simulink model "Joystick"  (R2018a)
settings: Solver=FixedStepDiscrete  StartTime=0.0  StopTime=inf  RelTol=1e-3  EnableMultiTasking=on
libraries: simulink x5, CustomLibrary x5
settings Model: SimulationMode=external  ExtModeTrigDuration=2  Creator=jonathancoulter  LastModifiedBy=jonathancoulter
settings SolverCC: AutoInsertRateTranBlk=on
settings OptimizationCC: DefaultParameterBehavior=Inlined  UseFloatMulNetSlope=on  InlineInvariantSignals=on  PassReuseOutputArgsThreshold=0  EfficientFloat2IntCast=on  MaxStackSize=64
settings DebuggingCC: ParameterTunabilityLossMsg=error
settings HardwareCC: ProdBitPerInt=16  ProdBitPerPointer=16  ProdBitPerSizeT=16  ProdBitPerPtrDiffT=16  ProdLargestAtomicFloat=None  ProdWordSize=8  ProdHWDeviceType=Atmel->AVR  UseEmbeddedCoderFeatures=off
settings SFSimCC: MATLABDynamicMemAlloc=off
settings RTWCC: SystemTargetFile=ert.tlc  HardwareBoard=Arduino Mega 2560  TLCOptions=-aInlineSetEventsForThisBaseRateFcn=TLC_FALSE -aSuppressMultiTaskScheduler=TLC_FALSE -aRateBasedStepFcn=1  TemplateMakefile=ert_default_tmf  Toolchain=Arduino AVR  BuildConfiguration=Faster Runs  CheckMdlBeforeBuild=Warning
settings CodeAppCC: ForceParamTrailComments=on  OperatorAnnotations=on  StateflowObjectComments=on  MATLABSourceComments=on
settings ERTTargetCC: ERTCustomFileBanners=off  SupportNonFinite=off  SupportContinuousTime=on  SupportNonInlinedSFcns=on  RemoveResetFunc=off  SupportVariableSizeSignals=on  ModelStepFunctionPrototypeControlCompliant=off  InlinedParameterPlacement=NonHierarchical

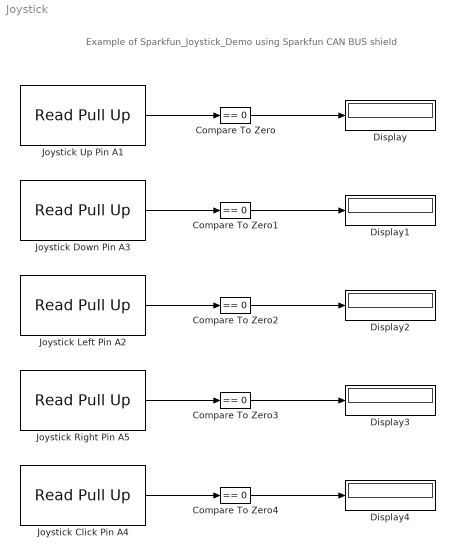
== system Joystick ==
  note: Example of Sparkfun_Joystick_Demo using Sparkfun CAN BUS shield
  Compare To Zero{,1..4} (5 alike) : simulink/Logic and Bit Operations/Compare To Zero  relop===  OutDataTypeStr=boolean
  Display{,1..4} (5 alike) : Display
  Joystick Click Pin A4 : CustomLibrary/Read Pull Up  pinNumberMask=58  SampleTimeMask=0.1
      settings: SourceProductName=Custom Blocks
  Joystick Down Pin A3 : CustomLibrary/Read Pull Up  pinNumberMask=57  SampleTimeMask=0.1
      settings: SourceProductName=Custom Blocks
  Joystick Left Pin A2 : CustomLibrary/Read Pull Up  pinNumberMask=56  SampleTimeMask=0.1
      settings: SourceProductName=Custom Blocks
  Joystick Right Pin A5 : CustomLibrary/Read Pull Up  pinNumberMask=59  SampleTimeMask=0.1
      settings: SourceProductName=Custom Blocks
  Joystick Up Pin A1 : CustomLibrary/Read Pull Up  pinNumberMask=55  SampleTimeMask=0.1
      settings: SourceProductName=Custom Blocks
  wires:
  Joystick Up Pin A1/1 -> Compare To Zero/1
  Joystick Down Pin A3/1 -> Compare To Zero1/1
  Joystick Left Pin A2/1 -> Compare To Zero2/1
  Joystick Right Pin A5/1 -> Compare To Zero3/1
  Joystick Click Pin A4/1 -> Compare To Zero4/1
  Compare To Zero/1 -> Display/1
  Compare To Zero1/1 -> Display1/1
  Compare To Zero2/1 -> Display2/1
  Compare To Zero3/1 -> Display3/1
  Compare To Zero4/1 -> Display4/1
